simulink model "Torque_Control"  (R2019b)
settings: Solver=VariableStepAuto  StartTime=0.0  StopTime=3  RelTol=1e-3
values from neighbouring files (symbols this model uses):
  ADAMS_communication_interval = 0.005    [Controls_Plant_1.m]    (also in Controls_Plant_3.m; Controls_Plant_5.m)
  ADAMS_communications_per_output_step = 1    [Controls_Plant_1.m]    (also in Controls_Plant_3.m; Controls_Plant_5.m)
  ADAMS_cwd = 'C:\Users\Justin\Documents\EMARO+\Centrale Nantes\Courses\AMORO\Lab\Lab 4'    [Controls_Plant_1.m]    (also in Controls_Plant_3.m; Controls_Plant_5.m)
  ADAMS_exec = ''    [Controls_Plant_1.m]    (also in Controls_Plant_3.m; Controls_Plant_5.m)
  ADAMS_host = 'LAPTOP-CH4PO0JS'    [Controls_Plant_1.m]    (also in Controls_Plant_3.m; Controls_Plant_5.m)
  ADAMS_init = ''    [Controls_Plant_1.m]    (also in Controls_Plant_3.m; Controls_Plant_5.m)
  ADAMS_inputs = 'dummy_input'    [Controls_Plant_1.m]    (also in Controls_Plant_3.m = 'q1d!q2d'; Controls_Plant_5.m = 'f1!f2')
  ADAMS_outputs = 'x!y!xd!yd!xdd!ydd!phi1!phi2!phi1d!phi2d!phi1dd!phi2dd!f1!f2'    [Controls_Plant_1.m]    (also in Controls_Plant_3.m = 'q1!q2'; Controls_Plant_5.m = 'q1!q2')
  ADAMS_prefix = 'Controls_Plant_1'    [Controls_Plant_1.m]    (also in Controls_Plant_3.m = 'Controls_Plant_3'; Controls_Plant_5.m = 'Controls_Plant_5')
  ADAMS_static = 'no'    [Controls_Plant_1.m]    (also in Controls_Plant_3.m; Controls_Plant_5.m)
  ADAMS_sysdir = 'C:\PROGRA~1\MSC~1.SOF\ADAMSS~1\2020_1\'    [Controls_Plant_1.m]    (also in Controls_Plant_3.m; Controls_Plant_5.m)
  ADAMS_time_offset = 0.0    (= 0)    [Controls_Plant_1.m]    (also in Controls_Plant_3.m; Controls_Plant_5.m)
settings Model: Creator=Justin  LastModifiedBy=Justin
settings SolverCC: AlgebraicLoopSolver=LineSearch

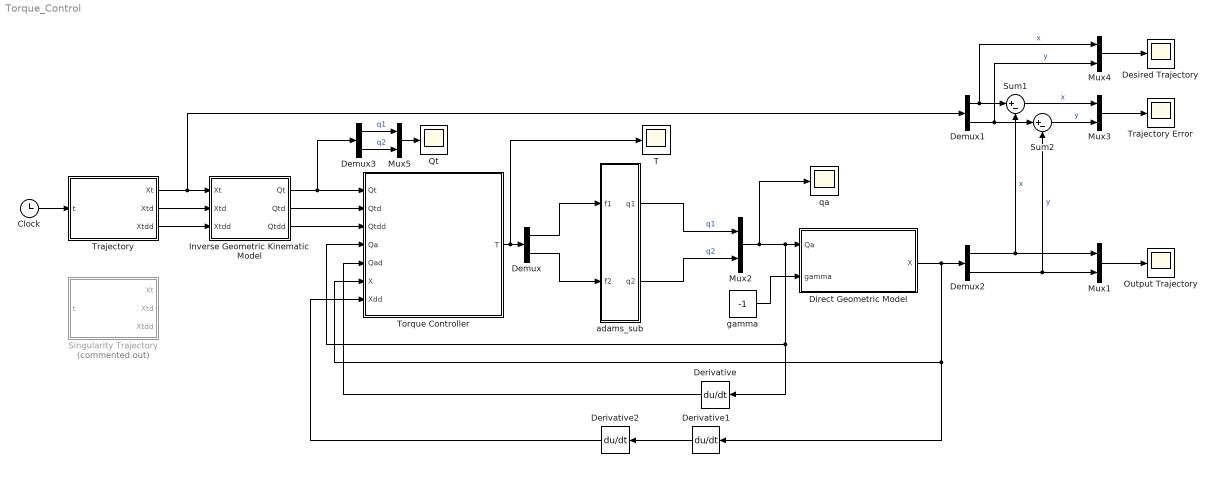
== system Torque_Control ==
  Clock : Clock
  Demux{,1..3} (4 alike) : Demux  Outputs=2
  Derivative : Derivative
  Derivative1 : Derivative
  Derivative2 : Derivative
  Desired Trajectory : Scope
  Direct Geometric Model : MATLAB Function  TreatAsAtomicUnit=on
  Inverse Geometric Kinematic Model : MATLAB Function  TreatAsAtomicUnit=on
  Mux{1..5} (5 alike) : Mux  Inputs=2
  Output Trajectory : Scope
  Qt : Scope
  Singularity Trajectory : MATLAB Function  Commented=on  TreatAsAtomicUnit=on
  Sum1 : Sum  Inputs=|+-
  Sum2 : Sum  Inputs=|+-
  T : Scope
  Torque Controller : MATLAB Function  TreatAsAtomicUnit=on
  Trajectory : MATLAB Function  TreatAsAtomicUnit=on
  Trajectory Error : Scope
  adams_sub : Subsystem
  gamma : Constant  Value=-1
  qa : Scope
  wires:
  gamma/1 -> Direct Geometric Model/2(gamma)
  adams_sub/2(q2) -> Mux2/2  "q2"
  adams_sub/1(q1) -> Mux2/1  "q1"
  Demux/1 -> adams_sub/1(f1)
  Demux/2 -> adams_sub/2(f2)
  Inverse Geometric Kinematic Model/2(Qtd) -> Torque Controller/2(Qtd)
  Inverse Geometric Kinematic Model/3(Qtdd) -> Torque Controller/3(Qtdd)
  Mux3/1 -> Trajectory Error/1
  Direct Geometric Model/1(X) -> Demux2/1, Torque Controller/6(X), Derivative1/1
  Torque Controller/1(T) -> T/1, Demux/1
  Derivative/1 -> Torque Controller/5(Qad)
  Derivative1/1 -> Derivative2/1
  Derivative2/1 -> Torque Controller/7(Xdd)
  Inverse Geometric Kinematic Model/1(Qt) -> Torque Controller/1(Qt), Demux3/1
  Demux1/1 -> Mux4/1, Sum1/1  "x"
  Demux2/1 -> Mux1/1, Sum1/2  "x"
  Demux2/2 -> Sum2/2, Mux1/2  "y"
  Sum2/1 -> Mux3/2  "y"
  Sum1/1 -> Mux3/1  "x"
  Mux1/1 -> Output Trajectory/1
  Mux4/1 -> Desired Trajectory/1
  Demux1/2 -> Mux4/2, Sum2/1  "y"
  Mux2/1 -> qa/1, Derivative/1, Torque Controller/4(Qa), Direct Geometric Model/1(Qa)
  Mux5/1 -> Qt/1
  Demux3/1 -> Mux5/1  "q1"
  Demux3/2 -> Mux5/2  "q2"
  Trajectory/1(Xt) -> Demux1/1, Inverse Geometric Kinematic Model/1(Xt)
  Trajectory/2(Xtd) -> Inverse Geometric Kinematic Model/2(Xtd)
  Trajectory/3(Xtdd) -> Inverse Geometric Kinematic Model/3(Xtdd)
  Clock/1 -> Trajectory/1(t)

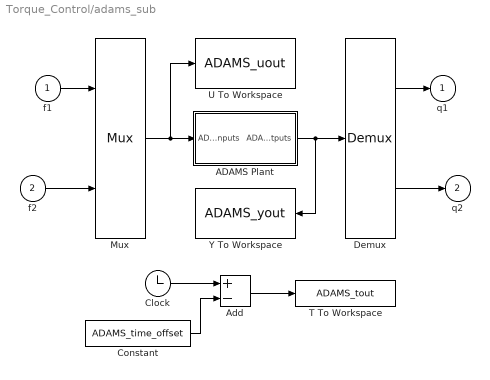
== system Torque_Control/adams_sub ==
  f1 : Inport
  f2 : Inport  Port=2
  ADAMS Plant : Subsystem  LoadFcn=|  InitFcn=clear mex  mask(Adams Plant){exevie=ADAMS_sysdir, nam_in=ADAMS_inputs, namout=ADAMS_outputs, nampre=ADAMS_prefix, outfil=ADAMS_prefix, exesol=ADAMS_exec, stat=ADAMS_static, inicmd=[ADAMS_init], exetyp=C++, comtyp=PIPE(DDE), workdir=ADAMS_cwd, ada_host=ADAMS_host, modani=batch, modsim=discrete, dft=no, simulink_lead_cosim=yes, pin_interp_order=0, pout_extrap_order=0, pin_extrap_order=0, pout_interp_order=0, dt_out=ADAMS_communication_interval, o_rate=ADAMS_communications_per_output_step, time_offset=ADAMS_time_offset, more=off}
      | %check based on dialog box setting for when setting by popup menu                                             
      | if exist('ADAMS_solver_type')                                                                                 
      |   if strcmp(ADAMS_solver_type,'C++')                                                                          
      |     set_param(gcb,'exetyp','C++');                                                                            
      |   else                                                                                                        
      |     set_param(gcb,'exetyp','Fortran');                                                                        
      |   end                                                                                                         
      | else                                                                                                          
      |   set_param(gcb,'exetyp','C++');                                                                              
      | end                                                                                                           
      | %set the mode if using acar_solver                                                                            
      | %REQUIRED HERE BECAUSE BELOW CAUSES MDLTERMINATE TO BE CALLED 2 TIMES IN MIDDLE OF SIMULATION WHEN SET IN MASK
      |                                                                                                               
      | %enable the direct feedthrough, sim mode, anim mode parameters by default                                     
      |                                                                                                               
      | if exist('set_some_params_states')                                                                            
      |                                                                                                               
      |   set_some_params_states({'dft','modsim','modani'},{'on','on','on'},'MaskEnables',gcb)                        
      |   %turn on direct feedthrough option                                                                          
      |   set_some_params_states({'dft'},{'on'},'MaskVisibilities',gcb)                                               
      |                                                                                                               
      |  end                                                                                                          
      |                                                                                                               
      |                                                                                                               
      | if exist('ADAMS_exec')                                                                                        
      |   if and(strcmp(get_param(gcb,'exesol'),'ADAMS_exec'),strcmp(ADAMS_exec,'acar_solver'))                       
      |     %set the sim mode to discrete -- only supported mode                                                      
      |     set_param(gcb,'modsim','discrete')                                                                        
      |      %turn off direct feedthrough option                                                                      
      |      set_some_params_states({'dft'},{'off'},'MaskVisibilities',gcb)                                           
      |     %set the animation mode to batch -- only supported mode                                                   
      |     set_param(gcb,'modani','batch')                                                                           
      |     %disable the direct feedthrough, sim mode, anim mode parameters                                           
      |     set_some_params_states({'modsim','modani'},{'off','off'},'MaskEnables',gcb)                               
      |   end
      |   if and(strcmp(get_param(gcb,'exesol'),'ADAMS_exec'),strcmp(ADAMS_exec,'apre_solver'))                       
      |     %set the sim mode to discrete -- only supported mode                                                      
      |     set_param(gcb,'modsim','discrete')                                                                        
      |      %turn off direct feedthrough option                                                                      
      |      set_some_params_states({'dft'},{'off'},'MaskVisibilities',gcb)                                           
      |     %set the animation mode to batch -- only supported mode                                                   
      |     set_param(gcb,'modani','batch')                                                                           
      |     %disable the direct feedthrough, sim mode, anim mode parameters                                           
      |     set_some_params_states({'modsim','modani'},{'off','off'},'MaskEnables',gcb)                               
      |   end                                                                                                  
      | end
      mask prompts: exevie "Adams install directory"; nam_in "Adams View input names"; namout "Adams View output names"; nampre "Adams model file prefix"; outfil "Output files prefix (opt.: if blank - no output)"; exesol "User executable (opt.: if blank - use standard)"; stat "Initial static simulation flag"; inicmd "Initialization commands"; exetyp "Adams Solver type"; comtyp "Interprocess option"; workdir "Adams working directory"; ada_host "Adams host"; modani "Animation mode"; modsim "Simulation mode"; dft "Direct feedthrough"; simulink_lead_cosim "Discrete Computational Order - Simulink Leads Adams"; pin_interp_order "Plant input interpolation order"; pout_extrap_order "Plant output extrapolation order"; pin_extrap_order "Plant input extrapolation order"; pout_interp_order "Plant output interpolation order"; dt_out "Communication interval"; o_rate "Number of communications per output step"; time_offset "Offset between Simulink and Adams simulation time"; more "More parameters"
      mask help: Simulate any Adams plant model either in Adams Solver form (.adm file) or in Adams View form (.cmd file)
      settings: OpenFcn=|
      | open_system(gcb,'mask')
      | if not(exist('set_some_params_states'))
      | 
      | warning('The script "set_some_params_states.m" cannot be found in the MATLAB PATH.  Cannot update the ADAMS Plant S-Function parameters.')
      | 
      | warning('Recommended action(optional):  run the Adams Controls .m file first to help choose the correct settings in the Adams S-Function block.')
      | 
      | end
      mask Help:
      | <html>
      | This S-Function represents the non-linear Adams Plant with the inputs sent to the Adams model as input #1 and Time as input #2<br>
      |  and the outputs generated by the Adams model.  See the Adams Controls documentation for more <br>
      | information.  This plant uses the following variables:<br>
      | <br>
      | <b>ADAMS_sysdir:</b> Adams installation directory<br>
      | <b>ADAMS_inputs:</b> Input variables View names vector<br>
      | <b>ADAMS_outputs :</b> Outputs variables View names vector<br>
      | <b>ADAMS_prefix:</b> ADAMS model files prefix (.adm, .cmd); also doubles as output files prefix<br>
      | <b>ADAMS_exec:</b>  Adams Solver user library or keyword (e.g., acar_solver)<br>
      | <b>ADAMS_static:</b> yes|no - initial static before Co-simulation(discrete)/Function Evaluation(continuous)<br>
      | <b>ADAMS_init:</b> Initialization commands (i.e., Adams View or Solver commands, depending on setting for Animation mode)<br>
      | <b>ADAMS_cwd:</b> Current working directory (for TCP/IP)<br>
      | <b>ADAMS_host:</b> Name of Adams server host (for TCP/IP)<br>
      | <b>ADAMS_mode:</b> Linear or non-linear (i.e., co-sim, function eval)<br>
      | <b>ADAMS_solver_type:</b> Fortran or C++ (used to set popup menu when first loaded)<br>
      | <b>ADAMS_communication_interval:</b> Time step at which Co-simulation exchange information (e.g.,0.005); also controls <br>output for continuous mode (Function Evaluation)<br>
      | <b>ADAMS_communications_per_output_step: </b>Sets Adams output rate (.res, .req, .gra) integer value (default: 1)<br>
      | <b>ADAMS_time_offset: </b>Removes this time offset from simulation time used by Adams. Adams will be sent a time value being Simulink simulation time - this value. (default: 0). Eg. if ADAMS_time_offset=2: if Simulink time=2 then Adams time = 0. Make sure that the Adams block is disabled when the Adams time is <0. If not an error will be raised. <br>
      | 
      | 
      | <br>
      | The following settings can be chosen:<br>
      | <br>
      | <b>Adams Solver type:</b>  Fortran or C++ (will also set ADAMS_solver_type)<br>
      | <b>Interprocess option:</b> Pipe(DDE), TCP/IP or DIRECT; TCP/IP can allow different machines run Adams and MATLAB<br>
      | <b>Animation mode:</b> batch (Solver, uses .adm) or interactive (View, uses .cmd)<br>
      | <b>Simulation mode:</b> discrete (Co-simulation) or continuous (Function Evaluation)<br>
      | <b>Discrete Computational Order - Simulink Lead Adams:</b> for discrete mode, chooses if Simulink leads the integration (yes) or lags (no);<br> if set to "no", can remove algebraic loop<br>
      | <b>Plant input interpolation order:</b> 0 = zero-order hold; 1 = linear (discrete mode only, where Simulink leads)<br>
      | <b>Plant output extrapolation order:</b> 0 = zero-order hold;1 = linear(discrete mode only, where Simulink leads)<br>
      | <b>Plant input extrapolation order:</b> 0 = zero-order hold; 1 = linear (discrete mode only, where Adams leads)<br>
      | <b>Plant output interpolation order:</b> 0 = zero-order hold;1 = linear(discrete mode only, where Adams leads)<br>
      | <b>Direct feedthrough:</b> yes|no - yes = Input directly effect output(continuous mode-only)<br>
      | 
      | </html>
      mask Callback exesol:
      | if exist('set_some_params_states')
      | %enable the direct feedthrough, sim mode, anim mode parameters
      | set_some_params_states({'dft','modsim','modani'},{'on','on','on'},'MaskEnables',gcb)
      | %turn on direct feedthrough option
      | set_some_params_states({'dft'},{'on'},'MaskVisibilities',gcb)
      | end
      | 
      | if exist('ADAMS_exec')
      |   if and(strcmp(get_param(gcb,'exesol'),'ADAMS_exec'),strcmp(ADAMS_exec,'acar_solver'))
      |     %set the sim mode to discrete -- only supported mode
      |     %REMOVED:  BELOW CAUSES MDLTERMINATE TO BE CALLED 2 TIMES IN MIDDLE OF SIMULATION
      |     %Now in LoadFcn callback
      |     %set_param(gcb,'modsim','discrete')
      |      %turn off direct feedthrough option
      |     set_some_params_states({'dft'},{'off'},'MaskVisibilities',gcb)
      |     %set the animation mode to batch -- only supported mode
      |     %REMOVED:  BELOW CAUSES MDLTERMINATE TO BE CALLED 2 TIMES IN MIDDLE OF SIMULATION
      |     %Now in LoadFcn callback
      |     %set_param(gcb,'modani','batch')
      |     %disable the direct feedthrough, sim mode, anim mode parameters
      |     set_some_params_states({'modsim','modani'},{'off','off'},'MaskEnables',gcb)
      |   end
      | end
      mask TypeOptions exetyp: Fortran | C++
      mask Callback exetyp:
      | if strcmp(get_param(gcb,'exetyp'),'C++')
      |     ADAMS_solver_type='C++';
      | else
      |     ADAMS_solver_type='Fortran';
      | end
      mask TypeOptions comtyp: PIPE(DDE) | TCP/IP | DIRECT
      mask Callback comtyp:
      | if exist('set_some_params_states')
      | if strcmp(get_param(gcb,'comtyp'),'PIPE(DDE)') || strcmp(get_param(gcb,'comtyp'),'DIRECT')
      |     %turn off cwd, host options
      |     set_some_params_states({'ada_host','workdir'},{'off','off'},'MaskVisibilities',gcb)
      | else%if strcmp(get_param(gcb,'modsim'),'TCP/IP')
      |     %turn on cwd, host options
      |     set_some_params_states({'ada_host','workdir'},{'on','on'},'MaskVisibilities',gcb)
      | end
      | end
      mask TypeOptions modani: batch | interactive
      mask TypeOptions modsim: discrete | continuous
      mask Callback modsim:
      | if exist('set_some_params_states')
      | if strcmp(get_param(gcb,'modsim'),'discrete')
      |      %turn off direct feedthrough option
      |     set_some_params_states({'dft'},{'off'},'MaskVisibilities',gcb)
      |     %turn on discrete co-sim type if want to see more
      |     if strcmp(get_param(gcb,'more'),'on')
      |         set_some_params_states({'simulink_lead_cosim'},{'on'},'MaskVisibilities',gcb)
      |     end
      |     if strcmp(get_param(gcb,'simulink_lead_cosim'),'yes')
      |         %turn on interpolation/extrapolation options
      |         set_some_params_states({'pin_interp_order','pout_extrap_order',},{'on','on'},'MaskVisibilities',gcb)
      |     else
      |         set_some_params_states({'pin_extrap_order','pout_interp_order'},{'on','on'},'MaskVisibilities',gcb)
      |     end
      | else%if strcmp(get_param(gcb,'modsim'),'continuous')
      |      %turn off direct feedthrough option
      |     set_some_params_states({'dft'},{'on'},'MaskVisibilities',gcb)
      |     %turn off interpolation/extrapolation options
      |     set_some_params_states({'pin_interp_order','pout_extrap_order','pin_extrap_order','pout_interp_order','simulink_lead_cosim'},{'off','off','off','off','off'},'MaskVisibilities',gcb)
      | end
      | end
      mask TypeOptions dft: no | yes
      mask TypeOptions simulink_lead_cosim: yes | no
      mask Callback simulink_lead_cosim:
      | if exist('set_some_params_states')
      | if (strcmp(get_param(gcb,'simulink_lead_cosim'),'yes') && strcmp(get_param(gcb,'modsim'),'discrete'))
      |      %turn off unused interpolate/extrapolate options
      |     set_some_params_states({'pin_extrap_order','pout_interp_order'},{'off','off'},'MaskVisibilities',gcb)
      |     %turn on used interpolate/extrapolate options
      |     set_some_params_states({'pin_interp_order','pout_extrap_order'},{'on','on'},'MaskVisibilities',gcb)
      | elseif (strcmp(get_param(gcb,'simulink_lead_cosim'),'no') && strcmp(get_param(gcb,'modsim'),'discrete'))
      |     %turn on used interpolate/extrapolate options
      |     set_some_params_states({'pin_extrap_order','pout_interp_order'},{'on','on'},'MaskVisibilities',gcb)
      |      %turn off unused interpolate/extrapolate options
      |     set_some_params_states({'pin_interp_order','pout_extrap_order'},{'off','off'},'MaskVisibilities',gcb)
      | end
      | end
      mask TypeOptions pin_interp_order: 0 | 1
      mask TypeOptions pout_extrap_order: 0 | 1
      mask TypeOptions pin_extrap_order: 0 | 1
      mask TypeOptions pout_interp_order: 0 | 1
      mask Callback more:
      | if exist('set_some_params_states')
      | if (strcmp(get_param(gcb,'more'),'on'))
      |      %turn on infrequently used options
      |     set_some_params_states({'exevie','nam_in','namout','exesol','stat','inicmd','time_offset'},{'on','on','on','on','on','on','on'},'MaskVisibilities',gcb)
      |     if strcmp(get_param(gcb,'modsim'),'discrete')
      |         set_some_params_states({'simulink_lead_cosim'},{'on'},'MaskVisibilities',gcb)
      |     end
      | elseif (strcmp(get_param(gcb,'more'),'off'))
      |     %turn off infrequently used options
      |     set_some_params_states({'exevie','nam_in','namout','exesol','stat','inicmd','time_offset'},{'off','off','off','off','off','off','off'},'MaskVisibilities',gcb)
      |     if strcmp(get_param(gcb,'modsim'),'discrete')
      |         set_some_params_states({'simulink_lead_cosim'},{'off'},'MaskVisibilities',gcb)
      |     end
      | end
      | end
      mask Display: disp( 'MSC Software' )
  Add : Sum  Inputs=+-
  Clock : Clock
  Constant : Constant  Value=ADAMS_time_offset
  Demux : Demux  Outputs=2
  Mux : Mux  Inputs=2
  T To Workspace : ToWorkspace  VariableName=ADAMS_tout
      settings: MaxDataPoints=100000
  U To Workspace : ToWorkspace  VariableName=ADAMS_uout
      settings: MaxDataPoints=100000
  Y To Workspace : ToWorkspace  VariableName=ADAMS_yout
      settings: MaxDataPoints=100000
  q1 : Outport
  q2 : Outport  Port=2
  wires:
  Mux/1 -> ADAMS Plant/1(ADAMS inputs), U To Workspace/1
  ADAMS Plant/1(ADAMS outputs) -> Demux/1, Y To Workspace/1
  Clock/1 -> Add/1
  Constant/1 -> Add/2
  Add/1 -> T To Workspace/1
  Demux/1 -> q1/1
  Demux/2 -> q2/1
  f1/1 -> Mux/1
  f2/1 -> Mux/2

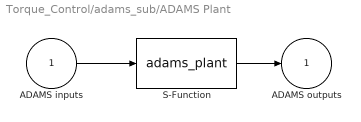
== system Torque_Control/adams_sub/ADAMS Plant ==
  ADAMS inputs : Inport
  S-Function : S-Function  StopFcn=clear mex  FunctionName=adams_plant  Parameters=exevie,exesol,stat,outfil,nampre,o_rate,nam_in,namout,dft,modsim,modani,dt_out,inicmd,exetyp,comtyp,ada_host, workdir,pin_interp_order,pout_extrap_order,pin_extrap_order,pout_interp_order,simulink_lead_cosim,time_offset  SFunctionDeploymentMode=off  EnableBusSupport=off
  ADAMS outputs : Outport  InitialOutput=0
  wires:
  ADAMS inputs/1 -> S-Function/1
  S-Function/1 -> ADAMS outputs/1

== matlab function Torque_Control/Singularity Trajectory ==
  data: Xt output; Xtd output; t input; Xtdd output
function [Xt,Xtd,Xtdd] = trajectory(t)
%Define parameters
xi = 0;
yi = 0.3;
xf = 0.15;
yf = -1.5;
tf1 = 3;
tf2 = 3;

%% Find Singularity Point
d = 0.4;
l = 0.3606;
gamma = -1;

q1 = 0;
q2 = gamma*sqrt(4*l^2 - d^2) + q1;

% Segments
OA = [d/2; q2];
AM = [-d; q1-q2]/2;
MC = gamma * real(sqrt(complex((4*l^2 - d^2 -(q1-q2)^2)/(d^2 + (q1-q2)^2)))) * [0 -1; 1 0] * AM;

Xs= OA + AM + MC;
xs = Xs(1);
ys = Xs(2);

if (t < tf1)
    %% Calculate path to singularity
    tf = tf1;
    % Calculate s, sd, and sdd equations
    s = 10*(t/tf)^3 - 15*(t/tf)^4 + 6*(t/tf)^5;

    sd = (30/tf)*(t/tf)^2 - (60/tf)*(t/tf)^3 + (30/tf)*(t/tf)^4;

    sdd = (60/tf)*(t/tf) - (180/tf)*(t/tf)^2 + (120/tf)*(t/tf)^3;

    %Calculate desired trajectory
    xt = xi + s*(xs-xi);
    yt = yi + s*(ys-yi);

    %Calculate desired velocity
    xtd = sd*(xs-xi);
    ytd = sd*(ys-yi);

    %Calculate desired acceleration
    xtdd = sdd*(xs-xi);
    ytdd = sdd*(ys-yi);
else 
%% Calculate path from singularity to final point
    tf = tf2;
    % Calculate s, sd, and sdd equations
    s = 10*((t-tf1)/tf)^3 - 15*((t-tf1)/tf)^4 + 6*((t-tf1)/tf)^5;
    
    sd = (30/tf)*((t-tf1)/tf)^2 - (60/tf)*((t-tf1)/tf)^3 + (30/tf)*((t-tf1)/tf)^4;
    
    sdd = (60/tf)*((t-tf1)/tf) - (180/tf)*((t-tf1)/tf)^2 + (120/tf)*((t-tf1)/tf)^3;
    
    %Calculate desired trajectory
    xt = xs + s*(xf-xs);
    yt = ys + s*(yf-ys);
    
    %Calculate desired velocity
    xtd = sd*(xf-xs);
    ytd = sd*(yf-ys);
    
    %Calculate desired acceleration
    xtdd = sdd*(xf-xs);
    ytdd = sdd*(yf-ys);
end
Xt = [xt;yt];
Xtd = [xtd;ytd];
Xtdd = [xtdd;ytdd];
end

== matlab function Torque_Control/Direct Geometric Model ==
  data: Qa input; X output; gamma input
function X = DGM(Qa,gamma)
    
    % Geometric parameters
    d = 0.4;
    l = 0.3606;
    
    q1 = Qa(1);
    q2 = Qa(2);
    
    % Segments
    OA = [d/2; q2];
    AM = [-d; q1-q2]/2;
    MC = gamma * sqrt((4*l^2 - d^2 -(q1-q2)^2)/(d^2 + (q1-q2)^2)) * [0 -1; 1 0] * AM;
    
    X= OA + AM + MC;
end

== matlab function Torque_Control/Trajectory ==
  data: Xt output; t input; Xtd output; Xtdd output
function [Xt,Xtd,Xtdd] = trajectory(t)
%% Initial Values
xi = 0;
yi = 0.3;
xf = 0.1;
yf = 0.5;
tf = 3;

%% Calculate S and S dot function
s = 10*(t/tf)^3 - 15*(t/tf)^4 + 6*(t/tf)^5;
sd = (30/tf)*(t/tf)^2 - (60/tf)*(t/tf)^3 + (30/tf)*(t/tf)^4;
sdd = (60/tf)*(t/tf) - (180/tf)*(t/tf)^2 + (120/tf)*(t/tf)^3;

%% Desired Trajectory
xt = xi + s*(xf-xi);
yt = yi + s*(yf-yi);
Xt = [xt;yt];

%% Desired Trajectory Velocity
xtd = sd*(xf-xi);
ytd = sd*(yf-yi);
Xtd = [xtd;ytd];

%% Desired Trajectory Acceleration
xtdd = sdd*(xf-xi);
ytdd = sdd*(yf-yi);
Xtdd = [xtdd;ytdd];
end

== matlab function Torque_Control/Inverse Geometric Kinematic Model ==
  data: Xt input; Qt output; Qtd output; Xtd input; Xtdd input; Qtdd output
function [Qt,Qtd,Qtdd]  = IGKM(Xt,Xtd,Xtdd)
%% Geometric Parameters
d= 0.4;
l= 0.3606;

%% Extract Parameters
x = Xt(1);
y = Xt(2);
xd = Xtd(1);
yd = Xtd(2);

%% Inverse Geometric Model
q1 = -sqrt(l^2 - (x + d/2)^2) + y;
q2 = -sqrt(l^2 - (x - d/2)^2) + y;
Qt = [q1;q2];

%% Inverse Kinematic Model
A = 2*[(x+d/2) (y-q1); (x-d/2) (y-q2)];
B = -2*[(y-q1) 0; 0 (y-q2)];

% Velocity of active joints from trajectory
Qtd = B\(-A*Xtd);
q1d = Qtd(1);
q2d = Qtd(2);

Ad = 2*[(xd) (yd-q1d); (xd) (yd-q2d)];
Bd = -2*[(yd-q1d) 0; 0 (yd-q2d)];

% Acceleration of active joints from trajectory
Qtdd = B\(-A*Xtdd - Ad*Xtd - Bd*Qtd);

end

== matlab function Torque_Control/Torque Controller ==
  data: Qt input; Qtd input; Qtdd input; Qa input; Qad input; T output; X input; Xdd input
function T = torqueController(Qt,Qtd,Qtdd,Qa,Qad,X,Xdd)

% M = mf
d = 0.4;
mp = 3;
mf = 1;

% Gains
Kp = 100;
Kd = 100;

% Extract Parameters
q1 = Qa(1);
q2 = Qa(2);
x = X(1);
y = X(2);
xdd = Xdd(1);
ydd = Xdd(2);

%Calculate Control Law based off equation T = M + c
A = 2*[(x + d/2) (y - q1) ; (x - d/2) (y - q2)];
B = -2*[(y - q1) 0 ; 0 (y-q2)]; 
J = -A\B;
c = J'*mp*[xdd ; ydd];

T = mf*(Qtdd + Kd*(Qtd - Qad) + Kp*(Qt - Qa)) + c;
end
